simulink model "gm_sampleModel1973_sub"  (R2023a)
settings: Solver=VariableStepAuto  StartTime=0.0  StopTime=10.0  RelTol=1e-3
libraries: simulink x4, hdlsllib x1
settings Model: Creator=user1  LastModifiedBy=user1
settings OptimizationCC: BlockReduction=off  ConditionallyExecuteInputs=off
settings DebuggingCC: InheritedTsInSrcMsg=none

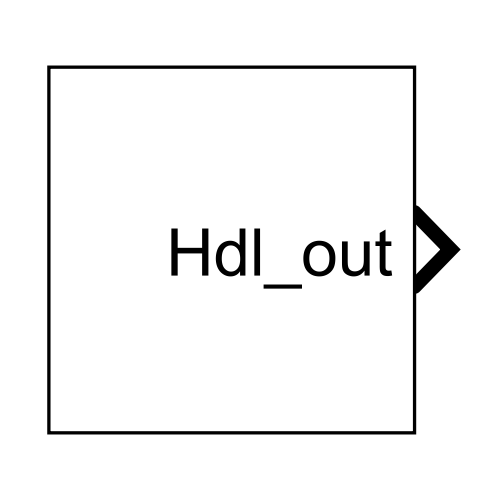
[thumbnail: Simulink's stored preview of the top-level diagram]
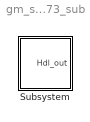
== system gm_sampleModel1973_sub ==
  Subsystem : Subsystem

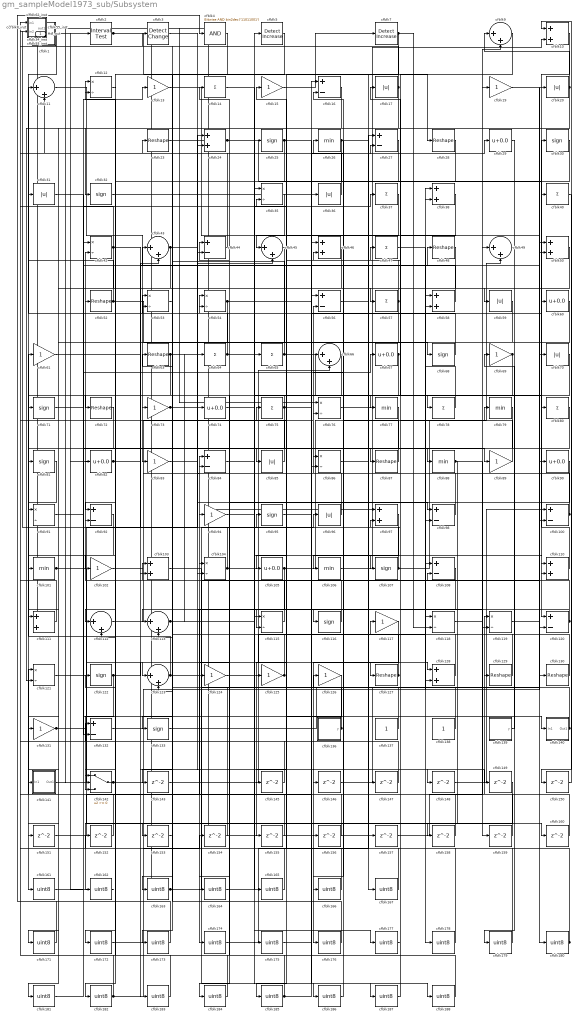
== system gm_sampleModel1973_sub/Subsystem ==
  cfblk1 : Subsystem  mask(Detect Fall Negative){vinit=double(0), InputProcessing=Elements as channels (sample based), OutDataTypeStr=uint8}
      mask prompts: vinit "Simulink:masks:InitialCondition_MP"; InputProcessing "Simulink:masks:InputProcessing_MP"; OutDataTypeStr "Simulink:masks:OutputDataType_MP"
      mask help: Simulink:masks:DetectFallNegative_MD
      mask init:
      | InputProcessing = 'Elements as channels (sample based)';
      | OutDataTypeStr = 'uint8';
      | vinit = double(0);
      mask TypeOptions InputProcessing: Simulink:masks:ColumnsAsChannelsFrameBased | Simulink:masks:ElementsAsChannelsSampleBased
      mask TypeOptions OutDataTypeStr: Simulink:masks:uint8 | Simulink:masks:boolean
      mask Display: fprintf('U < 0\n&  NOT\nU/z < 0')
  cfblk{10,24,38,46,50,58,97,103,110..111,128} (11 alike) : Sum  OutDataTypeStr=uint8
  cfblk{16,27,44,56,84,92,98,100,108,120,132} (11 alike) : Sum  Inputs=+-  OutDataTypeStr=uint8
  cfblk{26,77,79,88,101,106} (6 alike) : MinMax  OutDataTypeStr=uint8
  cfblk{13,15,19,61,69,73,83,89,94,102,117,124..126,131} (15 alike) : Gain  OutDataTypeStr=uint8
  cfblk{12,35,42,53..54,76,86,91,104,115,118..119,121} (13 alike) : Product  Inputs=*/  OutDataTypeStr=uint8  RndMeth=Zero  SaturateOnIntegerOverflow=on
  cfblk{29,60,67,74,82,90,105} (7 alike) : Bias  Bias=0.0  SaturateOnIntegerOverflow=off
  cfblk{25,30,32,68,71,81,95,107,116,122,133} (11 alike) : Signum
  cfblk{9,11,43,45,49,66,112..113,123} (9 alike) : Sum  Inputs=|++  OutDataTypeStr=uint8
  cfblk114_inst : Subsystem
  cfblk{23,28,48,52,63,72,87,127,129..130} (10 alike) : Reshape
  cfblk136 : Subsystem  mask(Counter Limited){uplimit=double(7), tsamp=double(-1)}
      mask prompts: uplimit "Simulink:masks:UpperLimit_MP"; tsamp "Simulink:masks:SampleTime_MP"
      mask help: Simulink:masks:CounterLimited_MD
      mask init:
      | nbits = double(8);
      | tsamp = double(-1);
      | uplimit = double(7);
  cfblk137 : Constant  OutDataTypeStr=uint8  SampleTime=-1
  cfblk138 : Constant  OutDataTypeStr=uint8  SampleTime=-1
  cfblk139 : Subsystem  mask(Counter Free-Running){NumBits=double(16), tsamp=double(-1)}
      mask prompts: NumBits "Simulink:masks:NumberOfBits_MP"; tsamp "Simulink:masks:SampleTime_MP"
      mask help: Simulink:masks:CounterFreeRunning_MD
  cfblk{14,37,40,47,57,64..65,75,78,80} (10 alike) : Sum  Inputs=+  OutDataTypeStr=uint8
  cfblk140 : Subsystem
  cfblk141 : Subsystem
  cfblk142 : Switch  OutDataTypeStr=uint8  SaturateOnIntegerOverflow=off  InputSameDT=off
  cfblk{143,145..160} (17 alike) : Delay  SampleTime=1
  cfblk{161..167,171..188} (25 alike) : DataTypeConversion  OutDataTypeStr=uint8  SaturateOnIntegerOverflow=off  RndMeth=Floor
  cfblk{17,20,31,36,59,70,85,96} (8 alike) : Abs  OutDataTypeStr=uint8  SaturateOnIntegerOverflow=off
  cfblk18_inst : Subsystem
  cfblk2 : hdlsllib/Logic and Bit Operations/Interval Test  IntervalClosedRight=on  uplimit=0.5  IntervalClosedLeft=on  lowlimit=-0.5  OutDataTypeStr=uint8
  cfblk21_inst : Subsystem
  cfblk3 : simulink/Logic and Bit Operations/Detect Change  vinit=0  OutDataTypeStr=uint8
      settings: LibrarySourceBlock=|
      | hdlsllib/Logic and Bit
      | Operations/Detect
      | Change
  cfblk34_inst : Subsystem
  cfblk4 : simulink/Logic and Bit Operations/Bitwise Operator  logicop=AND  UseBitMask=on  BitMask=bin2dec('11011001')  BitMaskRealWorld=Stored Integer
      settings: LibrarySourceBlock=|
      | hdlsllib/Logic and Bit
      | Operations/Bitwise
      | Operator
  cfblk5 : simulink/Logic and Bit Operations/Detect Increase  vinit=0.0  OutDataTypeStr=uint8
      settings: LibrarySourceBlock=|
      | hdlsllib/Logic and Bit
      | Operations/Detect
      | Increase
  cfblk55_inst : Subsystem
  cfblk62_inst : Subsystem
  cfblk7 : simulink/Logic and Bit Operations/Detect Increase  vinit=0.0  OutDataTypeStr=uint8
      settings: LibrarySourceBlock=|
      | hdlsllib/Logic and Bit
      | Operations/Detect
      | Increase
  cfblk8_inst : Subsystem
  cfblk93_inst : Subsystem
  Hdl_out : Outport  OutDataTypeStr=uint8  SampleTime=1
  wires:
  cfblk1/1(Y) -> cfblk161/1
  cfblk10/1 -> cfblk120/1
  cfblk100/1 -> cfblk56/2, cfblk56/1
  cfblk101/1 -> cfblk123/1, cfblk160/1
  cfblk102/1 -> cfblk76/2
  cfblk103/1 -> cfblk186/1
  cfblk104/1 -> cfblk66/2, cfblk18_inst/2(in2), cfblk128/1
  cfblk105/1 -> cfblk49/2, cfblk115/2
  cfblk106/1 -> cfblk10/2
  cfblk107/1 -> cfblk42/2, cfblk79/1
  cfblk108/1 -> cfblk174/1
  cfblk11/1 -> cfblk83/1
  cfblk110/1 -> cfblk30/1
  cfblk111/1 -> cfblk8_inst/1(in1)
  cfblk112/1 -> cfblk84/1
  cfblk113/1 -> cfblk148/1, cfblk64/1
  cfblk114_inst/1(out1) -> cfblk76/1
  cfblk115/1 -> cfblk82/1
  cfblk116/1 -> cfblk84/2
  cfblk117/1 -> cfblk176/1
  cfblk118/1 -> cfblk49/1
  cfblk119/1 -> cfblk20/1
  cfblk12/1 -> cfblk182/1
  cfblk120/1 -> cfblk92/2, cfblk113/1
  cfblk121/1 -> cfblk43/2
  cfblk122/1 -> cfblk142/3, cfblk127/1
  cfblk123/1 -> cfblk96/1, cfblk61/1
  cfblk124/1 -> cfblk155/1
  cfblk125/1 -> cfblk44/1, cfblk94/1
  cfblk126/1 -> cfblk185/1
  cfblk127/1 -> cfblk54/1, cfblk26/1
  cfblk128/1 -> cfblk15/1
  cfblk129/1 -> cfblk86/1
  cfblk13/1 -> cfblk180/1
  cfblk130/1 -> cfblk52/1
  cfblk131/1 -> cfblk74/1, cfblk2/1
  cfblk132/1 -> cfblk38/2
  cfblk133/1 -> cfblk70/1
  cfblk136/1(y) -> cfblk95/1, cfblk62_inst/2(in2)
  cfblk137/1 -> cfblk43/1
  cfblk138/1 -> cfblk38/1
  cfblk139/1(y) -> cfblk69/1
  cfblk14/1 -> cfblk187/1
  cfblk140/1(Out1) -> cfblk46/2, cfblk54/2
  cfblk141/1(Out1) -> cfblk24/2
  cfblk142/1 -> cfblk50/2, cfblk118/1
  cfblk143/1 -> cfblk98/2
  cfblk145/1 -> cfblk132/1
  cfblk146/1 -> cfblk58/2
  cfblk147/1 -> cfblk18_inst/1(in1)
  cfblk148/1 -> cfblk100/1
  cfblk149/1 -> cfblk162/1
  cfblk15/1 -> cfblk7/1
  cfblk150/1 -> cfblk10/1
  cfblk151/1 -> cfblk16/1
  cfblk152/1 -> cfblk21_inst/1(in1)
  cfblk153/1 -> cfblk53/1
  cfblk154/1 -> cfblk93_inst/2(in2)
  cfblk155/1 -> cfblk121/1
  cfblk156/1 -> cfblk103/1
  cfblk157/1 -> cfblk9/2
  cfblk158/1 -> cfblk104/1
  cfblk159/1 -> cfblk119/1
  cfblk16/1 -> cfblk121/2
  cfblk160/1 -> cfblk75/1
  cfblk161/1 -> cfblk67/1
  cfblk162/1 -> cfblk1/1(U)
  cfblk163/1 -> cfblk90/1, cfblk129/1, cfblk19/1
  cfblk164/1 -> cfblk5/1
  cfblk165/1 -> cfblk122/1
  cfblk166/1 -> cfblk55_inst/1(in1)
  cfblk167/1 -> cfblk55_inst/2(in2)
  cfblk17/1 -> cfblk34_inst/2(in2), cfblk32/1
  cfblk171/1 -> cfblk4/1
  cfblk172/1 -> cfblk108/1
  cfblk173/1 -> cfblk114_inst/2(in2)
  cfblk174/1 -> cfblk27/1
  cfblk175/1 -> cfblk27/2
  cfblk176/1 -> cfblk63/1
  cfblk177/1 -> cfblk117/1
  cfblk178/1 -> cfblk152/1
  cfblk179/1 -> cfblk47/1
  cfblk18_inst/1(out1) -> cfblk65/1
  cfblk180/1 -> cfblk93_inst/1(in1), cfblk113/2, cfblk35/2
  cfblk181/1 -> cfblk13/1
  cfblk182/1 -> cfblk21_inst/2(in2), cfblk154/1
  cfblk183/1 -> cfblk12/1
  cfblk184/1 -> cfblk12/2
  cfblk185/1 -> cfblk62_inst/1(in1), cfblk60/1, cfblk108/2
  cfblk186/1 -> cfblk126/1
  cfblk187/1 -> cfblk97/2
  cfblk188/1 -> cfblk14/1
  cfblk19/1 -> cfblk120/2
  cfblk2/1 -> cfblk28/1, cfblk167/1
  cfblk20/1 -> cfblk9/1, cfblk151/1
  cfblk21_inst/1(out1) -> cfblk142/2, cfblk111/2
  cfblk23/1 -> cfblk68/1
  cfblk24/1 -> cfblk130/1, cfblk40/1
  cfblk25/1 -> cfblk128/2, cfblk73/1
  cfblk26/1 -> cfblk44/2, cfblk116/1, cfblk110/2
  cfblk27/1 -> cfblk173/1
  cfblk28/1 -> cfblk72/1
  cfblk29/1 -> cfblk59/1
  cfblk3/1 -> cfblk98/1
  cfblk30/1 -> cfblk102/1
  cfblk31/1 -> cfblk89/1
  cfblk32/1 -> cfblk110/1
  cfblk34_inst/1(out1) -> cfblk91/2
  cfblk35/1 -> cfblk45/1
  cfblk36/1 -> cfblk34_inst/1(in1)
  cfblk37/1 -> cfblk145/1
  cfblk38/1 -> cfblk57/1
  cfblk4/1 -> cfblk172/1
  cfblk40/1 -> cfblk150/1
  cfblk42/1 -> cfblk8_inst/2(in2), cfblk111/1, cfblk146/1
  cfblk43/1 -> cfblk81/1, cfblk119/2
  cfblk44/1 -> cfblk11/2
  cfblk45/1 -> cfblk171/1
  cfblk46/1 -> cfblk112/2
  cfblk47/1 -> cfblk178/1
  cfblk48/1 -> cfblk143/1
  cfblk49/1 -> cfblk179/1
  cfblk5/1 -> cfblk163/1
  cfblk50/1 -> cfblk153/1
  cfblk52/1 -> cfblk175/1, cfblk11/1
  cfblk53/1 -> cfblk23/1
  cfblk54/1 -> cfblk133/1, cfblk107/1
  cfblk55_inst/1(out1) -> cfblk165/1
  cfblk56/1 -> cfblk29/1
  cfblk57/1 -> cfblk53/2, cfblk35/1, cfblk106/1
  cfblk58/1 -> cfblk42/1
  cfblk59/1 -> cfblk132/2
  cfblk60/1 -> cfblk166/1
  cfblk61/1 -> cfblk183/1
  cfblk62_inst/1(out1) -> cfblk97/1, cfblk157/1
  cfblk63/1 -> cfblk85/1, cfblk103/2
  cfblk64/1 -> cfblk31/1, cfblk86/2, cfblk78/1
  cfblk65/1 -> cfblk100/2, cfblk3/1
  cfblk66/1 -> cfblk131/1
  cfblk67/1 -> cfblk142/1, cfblk104/2
  cfblk68/1 -> cfblk16/2
  cfblk69/1 -> cfblk92/1, cfblk184/1
  cfblk7/1 -> cfblk125/1, cfblk118/2
  cfblk70/1 -> cfblk164/1
  cfblk71/1 -> cfblk140/1(In1)
  cfblk72/1 -> cfblk181/1
  cfblk73/1 -> cfblk45/2, cfblk123/2
  cfblk74/1 -> cfblk88/1
  cfblk75/1 -> cfblk71/1, cfblk188/1, cfblk101/1
  cfblk76/1 -> cfblk80/1
  cfblk77/1 -> cfblk87/1
  cfblk78/1 -> cfblk58/1
  cfblk79/1 -> cfblk105/1
  cfblk8_inst/1(out1) -> cfblk36/1
  cfblk80/1 -> cfblk112/1
  cfblk81/1 -> cfblk91/1
  cfblk82/1 -> cfblk48/1, Hdl_out/1
  cfblk83/1 -> cfblk149/1
  cfblk84/1 -> cfblk115/1
  cfblk85/1 -> cfblk114_inst/1(in1)
  cfblk86/1 -> cfblk147/1
  cfblk87/1 -> cfblk66/1
  cfblk88/1 -> cfblk159/1, cfblk158/1
  cfblk89/1 -> cfblk17/1
  cfblk9/1 -> cfblk77/1
  cfblk90/1 -> cfblk124/1
  cfblk91/1 -> cfblk37/1
  cfblk92/1 -> cfblk141/1(In1)
  cfblk93_inst/1(out1) -> cfblk25/1
  cfblk94/1 -> cfblk177/1
  cfblk95/1 -> cfblk50/1
  cfblk96/1 -> cfblk24/1
  cfblk97/1 -> cfblk156/1
  cfblk98/1 -> cfblk46/1

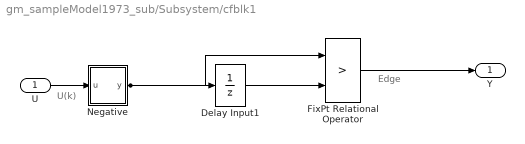
== system gm_sampleModel1973_sub/Subsystem/cfblk1 ==
  note: U(k)
  note: Edge
  U : Inport  OutDataTypeStr=uint8  SampleTime=1
  Delay Input1 : UnitDelay  Description=Store in Global RAM  DisableCoverage=on  InitialCondition=vinit  SampleTime=-1  HasFrameUpgradeWarning=on
  FixPt Relational Operator : RelationalOperator  Operator=>  OutDataTypeStr=fixdt(0, 8)  ZeroCross=off  InputSameDT=off
  Negative : Subsystem  mask(Compare To Zero){relop=<, OutDataTypeStr=boolean, ZeroCross=off}
      mask prompts: relop "Simulink:masks:Operator_MP"; OutDataTypeStr "Simulink:masks:OutputDataType_MP"; ZeroCross "Simulink:masks:EnableZerocrossingDetection_MP"
      mask help: Simulink:masks:CompareToZero_MD
      mask init:
      | OutDataTypeStr = 'boolean';
      | ZeroCross = 'off';
      | blkName = 'sampleModel1973_sub/Subsystem/cfblk1/Negative';
      | relop = '<';
      | setValue = 'boolean';
      mask TypeOptions relop: == | ~= | < | <= | >= | >
      mask TypeOptions OutDataTypeStr: Simulink:masks:uint8 | Simulink:masks:boolean
      mask Callback ZeroCross: sl('zeroCrossEnable', gcbh);
      mask Display: disp([relop,' 0'])
  Y : Outport  SampleTime=1
  wires:
  U/1 -> Negative/1(u)
  Delay Input1/1 -> FixPt Relational Operator/2
  FixPt Relational Operator/1 -> Y/1
  Negative/1(y) -> FixPt Relational Operator/1, Delay Input1/1

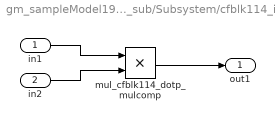
== system gm_sampleModel1973_sub/Subsystem/cfblk114_inst ==
  in1 : Inport  OutDataTypeStr=uint8  SampleTime=1
  in2 : Inport  Port=2  OutDataTypeStr=uint8  SampleTime=1
  mul_cfblk114_dotp_mulcomp : Product  Inputs=**  OutDataTypeStr=uint8  SampleTime=1
  out1 : Outport  OutDataTypeStr=uint8  SampleTime=1
  wires:
  in1/1 -> mul_cfblk114_dotp_mulcomp/1
  in2/1 -> mul_cfblk114_dotp_mulcomp/2
  mul_cfblk114_dotp_mulcomp/1 -> out1/1

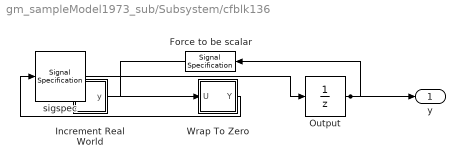
== system gm_sampleModel1973_sub/Subsystem/cfblk136 ==
  Force to be scalar : SignalSpecification  DisableCoverage=on  Dimensions=1
  Increment Real World : Subsystem  mask(Real World Value Increment){}
      mask help: Simulink:masks:RealWorldValueIncrement_MD
      mask Display: disp('V++')
  Output : UnitDelay  InitialCondition=0.0  SampleTime=tsamp  HasFrameUpgradeWarning=on
  Wrap To Zero : Subsystem  mask(Wrap To Zero){Threshold=double(7)}
      mask prompts: Threshold "Simulink:masks:Threshold_MP"
      mask help: Simulink:masks:WrapToZero_MD
  sigspec : SignalSpecification  OutDataTypeStr=uint8  Dimensions=1
  y : Outport  SampleTime=1
  wires:
  Force to be scalar/1 -> Increment Real World/1(u)
  Increment Real World/1(y) -> Wrap To Zero/1(U)
  Output/1 -> Force to be scalar/1, y/1
  Wrap To Zero/1(Y) -> sigspec/1
  sigspec/1 -> Output/1

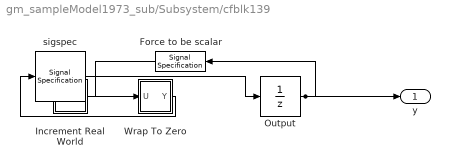
== system gm_sampleModel1973_sub/Subsystem/cfblk139 ==
  Force to be scalar : SignalSpecification  DisableCoverage=on  Dimensions=1
  Increment Real World : Subsystem  mask(Real World Value Increment){}
      mask help: Simulink:masks:RealWorldValueIncrement_MD
      mask Display: disp('V++')
  Output : UnitDelay  InitialCondition=0.0  SampleTime=tsamp  HasFrameUpgradeWarning=on
  Wrap To Zero : Subsystem  mask(Wrap To Zero){Threshold=double(65535)}
      mask prompts: Threshold "Simulink:masks:Threshold_MP"
      mask help: Simulink:masks:WrapToZero_MD
  sigspec : SignalSpecification  OutDataTypeStr=uint16  Dimensions=1
  y : Outport  SampleTime=1
  wires:
  Force to be scalar/1 -> Increment Real World/1(u)
  Increment Real World/1(y) -> Wrap To Zero/1(U)
  Output/1 -> Force to be scalar/1, y/1
  Wrap To Zero/1(Y) -> sigspec/1
  sigspec/1 -> Output/1

== system gm_sampleModel1973_sub/Subsystem/cfblk140 ==
  In1 : Inport  OutDataTypeStr=uint8  PortDimensions=1  SampleTime=1
  Out1 : Outport  SampleTime=1
  wires:
  In1/1 -> Out1/1

== system gm_sampleModel1973_sub/Subsystem/cfblk141 ==
  In1 : Inport  OutDataTypeStr=uint8  PortDimensions=1  SampleTime=1
  Out1 : Outport  SampleTime=1
  wires:
  In1/1 -> Out1/1

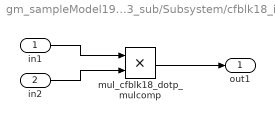
== system gm_sampleModel1973_sub/Subsystem/cfblk18_inst ==
  in1 : Inport  OutDataTypeStr=uint8  SampleTime=1
  in2 : Inport  Port=2  OutDataTypeStr=uint8  SampleTime=1
  mul_cfblk18_dotp_mulcomp : Product  Inputs=**  OutDataTypeStr=uint8  SampleTime=1
  out1 : Outport  OutDataTypeStr=uint8  SampleTime=1
  wires:
  in1/1 -> mul_cfblk18_dotp_mulcomp/1
  in2/1 -> mul_cfblk18_dotp_mulcomp/2
  mul_cfblk18_dotp_mulcomp/1 -> out1/1

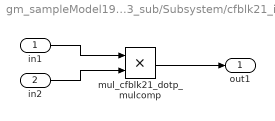
== system gm_sampleModel1973_sub/Subsystem/cfblk21_inst ==
  in1 : Inport  OutDataTypeStr=uint8  SampleTime=1
  in2 : Inport  Port=2  OutDataTypeStr=uint8  SampleTime=1
  mul_cfblk21_dotp_mulcomp : Product  Inputs=**  OutDataTypeStr=uint8  SampleTime=1
  out1 : Outport  OutDataTypeStr=uint8  SampleTime=1
  wires:
  in1/1 -> mul_cfblk21_dotp_mulcomp/1
  in2/1 -> mul_cfblk21_dotp_mulcomp/2
  mul_cfblk21_dotp_mulcomp/1 -> out1/1

== system gm_sampleModel1973_sub/Subsystem/cfblk34_inst ==
  in1 : Inport  OutDataTypeStr=uint8  SampleTime=1
  in2 : Inport  Port=2  OutDataTypeStr=uint8  SampleTime=1
  mul_cfblk34_dotp_mulcomp : Product  Inputs=**  OutDataTypeStr=uint8  SampleTime=1
  out1 : Outport  OutDataTypeStr=uint8  SampleTime=1
  wires:
  in1/1 -> mul_cfblk34_dotp_mulcomp/1
  in2/1 -> mul_cfblk34_dotp_mulcomp/2
  mul_cfblk34_dotp_mulcomp/1 -> out1/1

== system gm_sampleModel1973_sub/Subsystem/cfblk55_inst ==
  in1 : Inport  OutDataTypeStr=uint8  SampleTime=1
  in2 : Inport  Port=2  OutDataTypeStr=uint8  SampleTime=1
  mul_cfblk55_dotp_mulcomp : Product  Inputs=**  OutDataTypeStr=uint8  SampleTime=1
  out1 : Outport  OutDataTypeStr=uint8  SampleTime=1
  wires:
  in1/1 -> mul_cfblk55_dotp_mulcomp/1
  in2/1 -> mul_cfblk55_dotp_mulcomp/2
  mul_cfblk55_dotp_mulcomp/1 -> out1/1

== system gm_sampleModel1973_sub/Subsystem/cfblk62_inst ==
  in1 : Inport  OutDataTypeStr=uint8  SampleTime=1
  in2 : Inport  Port=2  OutDataTypeStr=uint8  SampleTime=1
  mul_cfblk62_dotp_mulcomp : Product  Inputs=**  OutDataTypeStr=uint8  SampleTime=1
  out1 : Outport  OutDataTypeStr=uint8  SampleTime=1
  wires:
  in1/1 -> mul_cfblk62_dotp_mulcomp/1
  in2/1 -> mul_cfblk62_dotp_mulcomp/2
  mul_cfblk62_dotp_mulcomp/1 -> out1/1

== system gm_sampleModel1973_sub/Subsystem/cfblk8_inst ==
  in1 : Inport  OutDataTypeStr=uint8  SampleTime=1
  in2 : Inport  Port=2  OutDataTypeStr=uint8  SampleTime=1
  mul_cfblk8_dotp_mulcomp : Product  Inputs=**  OutDataTypeStr=uint8  SampleTime=1
  out1 : Outport  OutDataTypeStr=uint8  SampleTime=1
  wires:
  in1/1 -> mul_cfblk8_dotp_mulcomp/1
  in2/1 -> mul_cfblk8_dotp_mulcomp/2
  mul_cfblk8_dotp_mulcomp/1 -> out1/1

== system gm_sampleModel1973_sub/Subsystem/cfblk93_inst ==
  in1 : Inport  OutDataTypeStr=uint8  SampleTime=1
  in2 : Inport  Port=2  OutDataTypeStr=uint8  SampleTime=1
  mul_cfblk93_dotp_mulcomp : Product  Inputs=**  OutDataTypeStr=uint8  SampleTime=1
  out1 : Outport  OutDataTypeStr=uint8  SampleTime=1
  wires:
  in1/1 -> mul_cfblk93_dotp_mulcomp/1
  in2/1 -> mul_cfblk93_dotp_mulcomp/2
  mul_cfblk93_dotp_mulcomp/1 -> out1/1

== system gm_sampleModel1973_sub/Subsystem/cfblk1/Negative ==
  u : Inport  OutDataTypeStr=uint8  SampleTime=1
  Compare : RelationalOperator  Operator=<  OutDataTypeStr=boolean  ZeroCross=off
  Constant : Constant  DisableCoverage=on  Value=0  OutDataTypeStr=Inherit: Inherit via back propagation  SampleTime=-1  PreserveConstantTs=on
  y : Outport  SampleTime=1
  wires:
  u/1 -> Compare/1
  Compare/1 -> y/1
  Constant/1 -> Compare/2

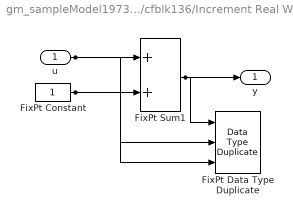
== system gm_sampleModel1973_sub/Subsystem/cfblk136/Increment Real World ==
  u : Inport  OutDataTypeStr=uint8  SampleTime=1
  FixPt Constant : Constant  DisableCoverage=on  OutDataTypeStr=Inherit: Inherit via back propagation  SampleTime=-1
  FixPt Data Type Duplicate : DataTypeDuplicate  DisableCoverage=on  NumInputPorts=3
  FixPt Sum1 : Sum  InputSameDT=on  OutDataTypeStr=Inherit: Inherit via back propagation  LockScale=on
  y : Outport  SampleTime=1
  wires:
  u/1 -> FixPt Sum1/1, FixPt Data Type Duplicate/2
  FixPt Constant/1 -> FixPt Sum1/2, FixPt Data Type Duplicate/3
  FixPt Sum1/1 -> FixPt Data Type Duplicate/1, y/1

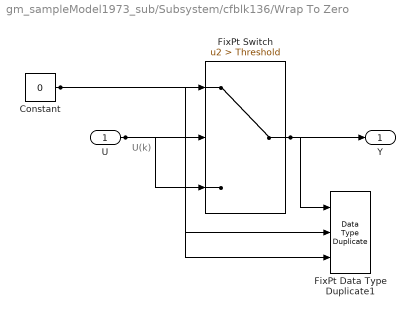
== system gm_sampleModel1973_sub/Subsystem/cfblk136/Wrap To Zero ==
  note: U(k)
  U : Inport  OutDataTypeStr=uint8  SampleTime=1
  Constant : Constant  DisableCoverage=on  Value=0  OutDataTypeStr=Inherit: Inherit via back propagation  SampleTime=-1
  FixPt Data Type Duplicate1 : DataTypeDuplicate  DisableCoverage=on  NumInputPorts=3
  FixPt Switch : Switch  Criteria=u2 > Threshold  Threshold=Threshold  OutDataTypeStr=Inherit: Inherit via back propagation  ZeroCross=off  SaturateOnIntegerOverflow=off  InputSameDT=off
  Y : Outport  SampleTime=1
  wires:
  U/1 -> FixPt Switch/3, FixPt Switch/2, FixPt Data Type Duplicate1/2
  Constant/1 -> FixPt Switch/1, FixPt Data Type Duplicate1/3
  FixPt Switch/1 -> FixPt Data Type Duplicate1/1, Y/1

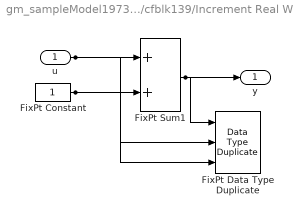
== system gm_sampleModel1973_sub/Subsystem/cfblk139/Increment Real World ==
  u : Inport  OutDataTypeStr=uint16  SampleTime=1
  FixPt Constant : Constant  DisableCoverage=on  OutDataTypeStr=Inherit: Inherit via back propagation  SampleTime=-1
  FixPt Data Type Duplicate : DataTypeDuplicate  DisableCoverage=on  NumInputPorts=3
  FixPt Sum1 : Sum  InputSameDT=on  OutDataTypeStr=Inherit: Inherit via back propagation  LockScale=on
  y : Outport  SampleTime=1
  wires:
  u/1 -> FixPt Sum1/1, FixPt Data Type Duplicate/2
  FixPt Constant/1 -> FixPt Sum1/2, FixPt Data Type Duplicate/3
  FixPt Sum1/1 -> FixPt Data Type Duplicate/1, y/1

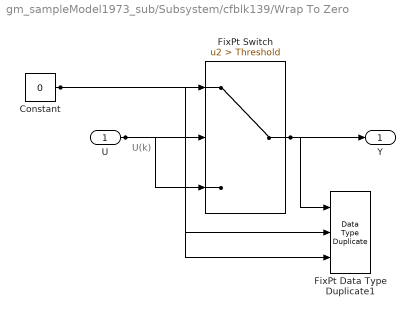
== system gm_sampleModel1973_sub/Subsystem/cfblk139/Wrap To Zero ==
  note: U(k)
  U : Inport  OutDataTypeStr=uint16  SampleTime=1
  Constant : Constant  DisableCoverage=on  Value=0  OutDataTypeStr=Inherit: Inherit via back propagation  SampleTime=-1
  FixPt Data Type Duplicate1 : DataTypeDuplicate  DisableCoverage=on  NumInputPorts=3
  FixPt Switch : Switch  Criteria=u2 > Threshold  Threshold=Threshold  OutDataTypeStr=Inherit: Inherit via back propagation  ZeroCross=off  SaturateOnIntegerOverflow=off  InputSameDT=off
  Y : Outport  SampleTime=1
  wires:
  U/1 -> FixPt Switch/3, FixPt Switch/2, FixPt Data Type Duplicate1/2
  Constant/1 -> FixPt Switch/1, FixPt Data Type Duplicate1/3
  FixPt Switch/1 -> FixPt Data Type Duplicate1/1, Y/1
